simulink model "hw5_sim"  (R2022b)
settings: Solver=VariableStepAuto  StartTime=0.0  StopTime=tspan  FixedStep=10  RelTol=1e-3
values from neighbouring files (symbols this model uses):
  epsilon_b_ECI_0 = [-.2; .4; .2]    [A421_FinalProject_Pt6.m]    (also in hw5.m)
  J = [812.04 0 0; 0 545.37 0; 0 0 627.71]    [A421_FinalProject_Pt5.m]    (also in A421_FinalProject_Pt6.m; Final_Project_Part_3_disturbances_torques.m; Final_Project_Pt4.m; hw5.m = diag([1200, 2000, 2800]))
  Kd = J*2*zeta*wn*[1;1;1]    [A421_FinalProject_Pt5.m]    (also in A421_FinalProject_Pt6.m = J*2*zeta*wn; hw5.m = J*2*zeta*wn.*eye(3))
  Kp = 2*J*wn^2*[1;1;1]    [A421_FinalProject_Pt5.m]    (also in A421_FinalProject_Pt6.m = 2*J*wn^2.; hw5.m = 2*J*wn^2*eye(3))
  q_b_ECI_0 = C2quat(C_b_ECI_0)    [A421_FinalProject_Pt5.m]    (also in A421_FinalProject_Pt6.m = [epsilon_b_ECI_0; sqrt(1-norm(epsilon_b_ECI_0)^2)]; Final_Project_Part_3_disturbances.m; Final_Project_Part_3_disturbances_init_Template-1.m; Final_Project_Part_3_disturbances_init_Template.m)
  q_C = [epsilon_C; sqrt(1-norm(epsilon_C)^2)]    [A421_FinalProject_Pt6.m]    (also in hw5.m)
  T = [0;0;0]    [A421_FinalProject_Pt6.m]    (also in hw5.m; main.m)
  w_b_ECI_0 = [0.001; -0.001; 0.002]    [A421_FinalProject_Pt5.m]    (also in A421_FinalProject_Pt6.m; Final_Project_Part_3_disturbances.m; Final_Project_Part_3_disturbances_init_Template-1.m; Final_Project_Part_3_disturbances_init_Template.m)
settings Model: Creator=emehiel  LastModifiedBy=ryanp
settings SolverCC: AlgebraicLoopSolver=TrustRegion
settings DebuggingCC: UnconnectedInputMsg=warning  UnconnectedOutputMsg=warning  UnconnectedLineMsg=warning  SFMachineParentedDataDiag=warning
settings ModelReferenceCC: EnableRefExpFcnMdlSchedulingChecks=on

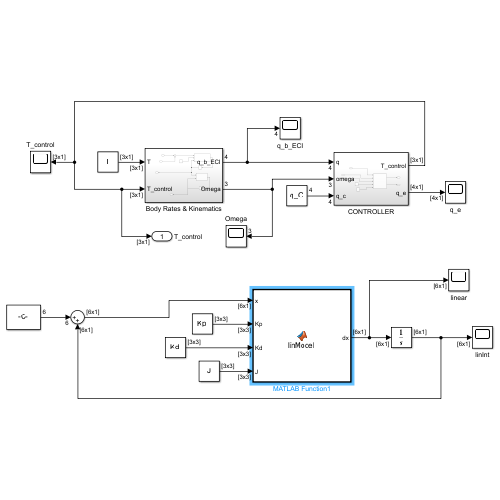
[thumbnail: Simulink's stored preview of the top-level diagram]
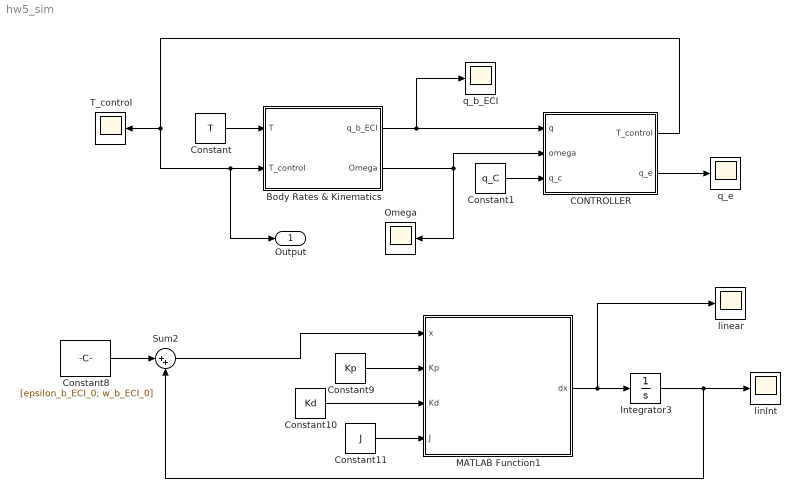
== system hw5_sim ==
  Body Rates & Kinematics : Subsystem
  CONTROLLER : Subsystem
  Constant : Constant  Value=T  VectorParams1D=off
  Constant1 : Constant  Value=q_C
  Constant10 : Constant  Value=Kd
  Constant11 : Constant  Value=J
  Constant8 : Constant  Value=[epsilon_b_ECI_0; w_b_ECI_0]
  Constant9 : Constant  Value=Kp
  Integrator3 : Integrator
  MATLAB Function1 : MATLAB Function  TreatAsAtomicUnit=on
  Omega : Scope
  Sum2 : Sum  Inputs=|++
  T_control : Scope
  linInt : Scope
  linear : Scope
  q_b_ECI : Scope
  q_e : Scope
  Output : Outport  SignalName=T_control
  wires:
  Body Rates & Kinematics/1(q_b_ECI) -> CONTROLLER/1(q), q_b_ECI/1
  Constant/1 -> Body Rates & Kinematics/1(T)
  CONTROLLER/1(T_control) -> Output/1, Body Rates & Kinematics/2(T_control), T_control/1
  Body Rates & Kinematics/2(Omega) -> CONTROLLER/2(omega), Omega/1
  CONTROLLER/2(q_e) -> q_e/1
  Constant1/1 -> CONTROLLER/3(q_c)
  Constant11/1 -> MATLAB Function1/4(J)
  Constant10/1 -> MATLAB Function1/3(Kd)
  Constant9/1 -> MATLAB Function1/2(Kp)
  MATLAB Function1/1(dx) -> linear/1, Integrator3/1
  Constant8/1 -> Sum2/1
  Sum2/1 -> MATLAB Function1/1(x)
  Integrator3/1 -> Sum2/2, linInt/1

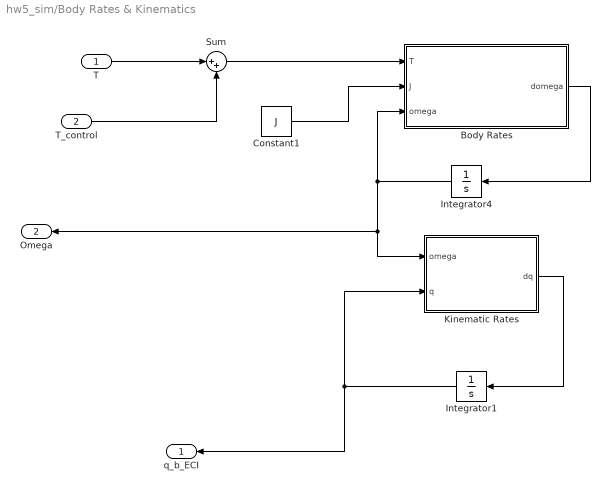
== system hw5_sim/Body Rates & Kinematics ==
  T : Inport
  T_control : Inport  Port=2
  Body Rates : MATLAB Function  TreatAsAtomicUnit=on
  Constant1 : Constant  Value=J
  Integrator1 : Integrator  InitialCondition=q_b_ECI_0
  Integrator4 : Integrator  InitialCondition=w_b_ECI_0
  Kinematic Rates : MATLAB Function  TreatAsAtomicUnit=on
  Sum : Sum  Inputs=|++
  q_b_ECI : Outport
  Omega : Outport  Port=2
  wires:
  Kinematic Rates/1(dq) -> Integrator1/1
  Integrator1/1 -> q_b_ECI/1, Kinematic Rates/2(q)
  Body Rates/1(domega) -> Integrator4/1
  Integrator4/1 -> Omega/1, Kinematic Rates/1(omega), Body Rates/3(omega)
  Constant1/1 -> Body Rates/2(J)
  T/1 -> Sum/1
  Sum/1 -> Body Rates/1(T)
  T_control/1 -> Sum/2

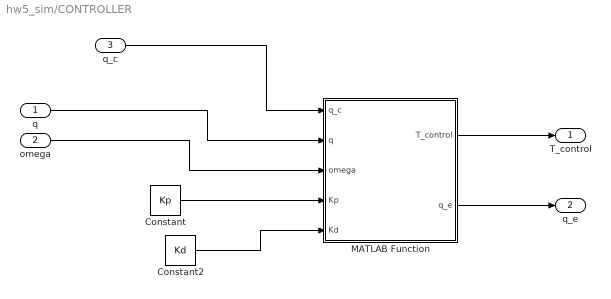
== system hw5_sim/CONTROLLER ==
  q : Inport
  omega : Inport  Port=2
  q_c : Inport  Port=3
  Constant : Constant  Value=Kp
  Constant2 : Constant  Value=Kd
  MATLAB Function : MATLAB Function  TreatAsAtomicUnit=on
  T_control : Outport
  q_e : Outport  Port=2
  wires:
  q/1 -> MATLAB Function/2(q)
  omega/1 -> MATLAB Function/3(omega)
  Constant/1 -> MATLAB Function/4(Kp)
  Constant2/1 -> MATLAB Function/5(Kd)
  MATLAB Function/2(q_e) -> q_e/1
  q_c/1 -> MATLAB Function/1(q_c)
  MATLAB Function/1(T_control) -> T_control/1

== matlab function hw5_sim/CONTROLLER/MATLAB Function ==
  data: q_c input; T_control output; q input; omega input; Kp input; Kd input; q_e output
function [T_control, q_e] = controller(q_c, q, omega, Kp, Kd)
%#codegen
% q_e = quatMult(q, quatConjugate(q_c));

% Quat conjugate rotated
q_c_conj = [q_c(1), -q_c(2), -q_c(3), -q_c(4)];
p0 = q_c_conj(1); p1 = q_c_conj(2); p2 = q_c_conj(3); p3 = q_c_conj(4);

% Quat multiplication
q0 = q(1,1); q1 = q(2); q2 = q(3); q3 = q(4);

q1 = q0 * p0 - q1 * p1 - q2 * p2 - q3 * p3;
q2 = q0 * p1 + q1 * p0 + q2 * p3 - q3 * p2;
q3 = q0 * p2 - q1 * p3 + q2 * p0 + q3 * p1;
q4 = q0 * p3 + q1 * p2 - q2 * p1 + q3 * p0;

q_e = [q1; q2; q3; q4];
disp(q_e)
% q_c

% T_control = -Kp*q_e(1:3,1) - Kd*omega;
T_control= 2*(-Kp*q_e(1:3) - Kd*omega);


end

== matlab function hw5_sim/MATLAB Function1 ==
  data: x input; Kp input; Kd input; J input; dx output
function dx = linModel(x, Kp, Kd, J)
    theta = x(1:3);  % Angular pos
    omega = x(4:6);  % Angular vel
    
    % PD Controller
    tau = -Kp *(theta -  [0; 0; 0]) - Kd*(omega - [0; 0; 0]);
    M = tau.*[2; 2; 2];
    
    alpha = J\(M- cross(omega, J*omega));

    dx = [omega; alpha];
end

== matlab function hw5_sim/Body Rates & Kinematics/Kinematic Rates ==
  data: omega input; q input; dq output
function dq  = kinematics(omega, q)
%#codegen

% I = eye(3); %Identity
% 
% unpack quaternion
% eps1 = q(1);
% eps2 = q(2);
% eps3 = q(3);
% eps = [eps1; eps2; eps3];
% 
% eda = q(4);
% 
% compute the derivative of the quaternion components here
%              
% Quaternion rates Eq.1.56
% eps_cross = [0,  -eps3, eps2;
%              eps3,  0, -eps1;
%              -eps2, eps1, 0];
% 
% deps = 0.5*(eda*I + eps_cross)*omega;
% deda = -0.5*eps'*omega;
% 
% dq = [deps; deda];
% 
% compute the derivative of the Euler Angle components here
%             
% Euler rates
% phi = E(1);
% theta = E(2);
% R = [1 sin(phi)*tan(theta) cos(phi)*tan(theta);
%      0     cos(phi)           -sin(phi);
%      0 sin(phi)*sec(theta) cos(phi)*sec(theta)];
%     
% dE = R*omega;
% unpack quaternion

epsilon = q(1:3,1);
eta = q(4,1);

% depsilon = 1/2*(eta*eye(3) + vect2cross(epsilon))*omega;
epsilon_cross = [0, -epsilon(3), epsilon(2);
                     epsilon(3), 0, -epsilon(1);
                     -epsilon(2), epsilon(1), 0];

% Compute depsilon
depsilon = 1/2 * (eta * eye(3) + epsilon_cross) * omega;
deta = -1/2*epsilon'*omega;

dq = [depsilon; deta];


end

== matlab function hw5_sim/Body Rates & Kinematics/Body Rates ==
  data: T input; J input; omega input; domega output
function domega = dynamics(T, J, omega)
%#codegen


% Compute the derivative of the angular velocity $\omega$ here

domega = J \ (T - cross(-omega, J*omega));

% phi = omega(1);
% theta = omega(2);
% psi = omega(3);
% 
% %From body to euler rates
% matrix = [1 sin(phi)*tan(theta) cos(phi)*tan(theta);
%           0    cos(phi)            -sin(phi);
%           0 sin(phi)*sec(theta) cos(phi)*sec(theta)];
% 
% domega = matrix * omega;

end
